simulink model "c00002M_harness"  (R2018a)
settings: Solver=FixedStepAuto  StartTime=0.0  StopTime=300  FixedStep=0.1  RelTol=1e-3
undefined symbols (not defined in the file): A1, hmax, R1, R2, sigbuilder_block, TempThreshold
(part 5 of 14)

== system c00002M_harness/M075/Tank3 ==
  CT3 : Inport
  MR3 : Inport  Port=2
  T3 : Inport  Port=3
  EB3 : Inport  Port=4
  Control : Subsystem
  Memory : Memory
  TankModel : Subsystem
  LL3 : Outport
  wires:
  TankModel/1(LiquidLevel) -> Memory/1, LL3/1
  Control/2(LiquidOut) -> TankModel/2(LiquidOut)
  Memory/1 -> Control/5(LiquidLevel)
  MR3/1 -> Control/2(ManualReference)
  CT3/1 -> Control/1(ControlType)
  EB3/1 -> Control/3(EmergencyButton)
  T3/1 -> Control/4(Temperature)
  Control/1(LiquidIn) -> TankModel/1(LiquidIn)

== system c00002M_harness/M076/Tank1 ==
  CT1 : Inport
  MR1 : Inport  Port=2
  T1 : Inport  Port=3
  EB1 : Inport  Port=4
  Control : Subsystem
  Memory : Memory
  TankModel : Subsystem
  LL1 : Outport
  wires:
  TankModel/1(LiquidLevel) -> Memory/1, LL1/1
  Control/2(LiquidOut) -> TankModel/2(LiquidOut)
  Memory/1 -> Control/5(LiquidLevel)
  MR1/1 -> Control/2(ManualReference)
  CT1/1 -> Control/1(ControlType)
  EB1/1 -> Control/3(EmergencyButton)
  T1/1 -> Control/4(Temperature)
  Control/1(LiquidIn) -> TankModel/1(LiquidIn)

== system c00002M_harness/M076/Tank3 ==
  CT3 : Inport
  MR3 : Inport  Port=2
  T3 : Inport  Port=3
  EB3 : Inport  Port=4
  Control : Subsystem
  Memory : Memory
  TankModel : Subsystem
  LL3 : Outport
  wires:
  TankModel/1(LiquidLevel) -> Memory/1, LL3/1
  Control/2(LiquidOut) -> TankModel/2(LiquidOut)
  Memory/1 -> Control/5(LiquidLevel)
  MR3/1 -> Control/2(ManualReference)
  CT3/1 -> Control/1(ControlType)
  EB3/1 -> Control/3(EmergencyButton)
  T3/1 -> Control/4(Temperature)
  Control/1(LiquidIn) -> TankModel/1(LiquidIn)

== system c00002M_harness/M077/Tank1 ==
  CT1 : Inport
  MR1 : Inport  Port=2
  T1 : Inport  Port=3
  EB1 : Inport  Port=4
  Control : Subsystem
  Memory : Memory
  TankModel : Subsystem
  LL1 : Outport
  wires:
  TankModel/1(LiquidLevel) -> Memory/1, LL1/1
  Control/2(LiquidOut) -> TankModel/2(LiquidOut)
  Memory/1 -> Control/5(LiquidLevel)
  MR1/1 -> Control/2(ManualReference)
  CT1/1 -> Control/1(ControlType)
  EB1/1 -> Control/3(EmergencyButton)
  T1/1 -> Control/4(Temperature)
  Control/1(LiquidIn) -> TankModel/1(LiquidIn)

== system c00002M_harness/M077/Tank3 ==
  CT3 : Inport
  MR3 : Inport  Port=2
  T3 : Inport  Port=3
  EB3 : Inport  Port=4
  Control : Subsystem
  Memory : Memory
  TankModel : Subsystem
  LL3 : Outport
  wires:
  TankModel/1(LiquidLevel) -> Memory/1, LL3/1
  Control/2(LiquidOut) -> TankModel/2(LiquidOut)
  Memory/1 -> Control/5(LiquidLevel)
  MR3/1 -> Control/2(ManualReference)
  CT3/1 -> Control/1(ControlType)
  EB3/1 -> Control/3(EmergencyButton)
  T3/1 -> Control/4(Temperature)
  Control/1(LiquidIn) -> TankModel/1(LiquidIn)

== system c00002M_harness/M078/Tank1 ==
  CT1 : Inport
  MR1 : Inport  Port=2
  T1 : Inport  Port=3
  EB1 : Inport  Port=4
  Control : Subsystem
  Memory : Memory
  TankModel : Subsystem
  LL1 : Outport
  wires:
  TankModel/1(LiquidLevel) -> Memory/1, LL1/1
  Control/2(LiquidOut) -> TankModel/2(LiquidOut)
  Memory/1 -> Control/5(LiquidLevel)
  MR1/1 -> Control/2(ManualReference)
  CT1/1 -> Control/1(ControlType)
  EB1/1 -> Control/3(EmergencyButton)
  T1/1 -> Control/4(Temperature)
  Control/1(LiquidIn) -> TankModel/1(LiquidIn)

== system c00002M_harness/M078/Tank3 ==
  CT3 : Inport
  MR3 : Inport  Port=2
  T3 : Inport  Port=3
  EB3 : Inport  Port=4
  Control : Subsystem
  Memory : Memory
  TankModel : Subsystem
  LL3 : Outport
  wires:
  TankModel/1(LiquidLevel) -> Memory/1, LL3/1
  Control/2(LiquidOut) -> TankModel/2(LiquidOut)
  Memory/1 -> Control/5(LiquidLevel)
  MR3/1 -> Control/2(ManualReference)
  CT3/1 -> Control/1(ControlType)
  EB3/1 -> Control/3(EmergencyButton)
  T3/1 -> Control/4(Temperature)
  Control/1(LiquidIn) -> TankModel/1(LiquidIn)

== system c00002M_harness/M079/Tank1 ==
  CT1 : Inport
  MR1 : Inport  Port=2
  T1 : Inport  Port=3
  EB1 : Inport  Port=4
  Control : Subsystem
  Memory : Memory
  TankModel : Subsystem
  LL1 : Outport
  wires:
  TankModel/1(LiquidLevel) -> Memory/1, LL1/1
  Control/2(LiquidOut) -> TankModel/2(LiquidOut)
  Memory/1 -> Control/5(LiquidLevel)
  MR1/1 -> Control/2(ManualReference)
  CT1/1 -> Control/1(ControlType)
  EB1/1 -> Control/3(EmergencyButton)
  T1/1 -> Control/4(Temperature)
  Control/1(LiquidIn) -> TankModel/1(LiquidIn)

== system c00002M_harness/M079/Tank3 ==
  CT3 : Inport
  MR3 : Inport  Port=2
  T3 : Inport  Port=3
  EB3 : Inport  Port=4
  Control : Subsystem
  Memory : Memory
  TankModel : Subsystem
  LL3 : Outport
  wires:
  TankModel/1(LiquidLevel) -> Memory/1, LL3/1
  Control/2(LiquidOut) -> TankModel/2(LiquidOut)
  Memory/1 -> Control/5(LiquidLevel)
  MR3/1 -> Control/2(ManualReference)
  CT3/1 -> Control/1(ControlType)
  EB3/1 -> Control/3(EmergencyButton)
  T3/1 -> Control/4(Temperature)
  Control/1(LiquidIn) -> TankModel/1(LiquidIn)

== system c00002M_harness/M080/Tank1 ==
  CT1 : Inport
  MR1 : Inport  Port=2
  T1 : Inport  Port=3
  EB1 : Inport  Port=4
  Control : Subsystem
  Memory : Memory
  TankModel : Subsystem
  LL1 : Outport
  wires:
  TankModel/1(LiquidLevel) -> Memory/1, LL1/1
  Control/2(LiquidOut) -> TankModel/2(LiquidOut)
  Memory/1 -> Control/5(LiquidLevel)
  MR1/1 -> Control/2(ManualReference)
  CT1/1 -> Control/1(ControlType)
  EB1/1 -> Control/3(EmergencyButton)
  T1/1 -> Control/4(Temperature)
  Control/1(LiquidIn) -> TankModel/1(LiquidIn)

== system c00002M_harness/M080/Tank3 ==
  CT3 : Inport
  MR3 : Inport  Port=2
  T3 : Inport  Port=3
  EB3 : Inport  Port=4
  Control : Subsystem
  Memory : Memory
  TankModel : Subsystem
  LL3 : Outport
  wires:
  TankModel/1(LiquidLevel) -> Memory/1, LL3/1
  Control/2(LiquidOut) -> TankModel/2(LiquidOut)
  Memory/1 -> Control/5(LiquidLevel)
  MR3/1 -> Control/2(ManualReference)
  CT3/1 -> Control/1(ControlType)
  EB3/1 -> Control/3(EmergencyButton)
  T3/1 -> Control/4(Temperature)
  Control/1(LiquidIn) -> TankModel/1(LiquidIn)

== system c00002M_harness/M081/Tank1 ==
  CT1 : Inport
  MR1 : Inport  Port=2
  T1 : Inport  Port=3
  EB1 : Inport  Port=4
  Control : Subsystem
  Memory : Memory
  TankModel : Subsystem
  LL1 : Outport
  wires:
  TankModel/1(LiquidLevel) -> Memory/1, LL1/1
  Control/2(LiquidOut) -> TankModel/2(LiquidOut)
  Memory/1 -> Control/5(LiquidLevel)
  MR1/1 -> Control/2(ManualReference)
  CT1/1 -> Control/1(ControlType)
  EB1/1 -> Control/3(EmergencyButton)
  T1/1 -> Control/4(Temperature)
  Control/1(LiquidIn) -> TankModel/1(LiquidIn)

== system c00002M_harness/M081/Tank3 ==
  CT3 : Inport
  MR3 : Inport  Port=2
  T3 : Inport  Port=3
  EB3 : Inport  Port=4
  Control : Subsystem
  Memory : Memory
  TankModel : Subsystem
  LL3 : Outport
  wires:
  TankModel/1(LiquidLevel) -> Memory/1, LL3/1
  Control/2(LiquidOut) -> TankModel/2(LiquidOut)
  Memory/1 -> Control/5(LiquidLevel)
  MR3/1 -> Control/2(ManualReference)
  CT3/1 -> Control/1(ControlType)
  EB3/1 -> Control/3(EmergencyButton)
  T3/1 -> Control/4(Temperature)
  Control/1(LiquidIn) -> TankModel/1(LiquidIn)

== system c00002M_harness/M082/Tank1 ==
  CT1 : Inport
  MR1 : Inport  Port=2
  T1 : Inport  Port=3
  EB1 : Inport  Port=4
  Control : Subsystem
  Memory : Memory
  TankModel : Subsystem
  LL1 : Outport
  wires:
  TankModel/1(LiquidLevel) -> Memory/1, LL1/1
  Control/2(LiquidOut) -> TankModel/2(LiquidOut)
  Memory/1 -> Control/5(LiquidLevel)
  MR1/1 -> Control/2(ManualReference)
  CT1/1 -> Control/1(ControlType)
  EB1/1 -> Control/3(EmergencyButton)
  T1/1 -> Control/4(Temperature)
  Control/1(LiquidIn) -> TankModel/1(LiquidIn)

== system c00002M_harness/M082/Tank3 ==
  CT3 : Inport
  MR3 : Inport  Port=2
  T3 : Inport  Port=3
  EB3 : Inport  Port=4
  Control : Subsystem
  Memory : Memory
  TankModel : Subsystem
  LL3 : Outport
  wires:
  TankModel/1(LiquidLevel) -> Memory/1, LL3/1
  Control/2(LiquidOut) -> TankModel/2(LiquidOut)
  Memory/1 -> Control/5(LiquidLevel)
  MR3/1 -> Control/2(ManualReference)
  CT3/1 -> Control/1(ControlType)
  EB3/1 -> Control/3(EmergencyButton)
  T3/1 -> Control/4(Temperature)
  Control/1(LiquidIn) -> TankModel/1(LiquidIn)

== system c00002M_harness/M165/Tank1 ==
  CT1 : Inport
  MR1 : Inport  Port=2
  T1 : Inport  Port=3
  EB1 : Inport  Port=4
  Control : Subsystem
  Memory : Memory
  TankModel : Subsystem
  LL1 : Outport
  wires:
  TankModel/1(LiquidLevel) -> Memory/1, LL1/1
  Control/2(LiquidOut) -> TankModel/2(LiquidOut)
  Memory/1 -> Control/5(LiquidLevel)
  MR1/1 -> Control/2(ManualReference)
  CT1/1 -> Control/1(ControlType)
  EB1/1 -> Control/3(EmergencyButton)
  T1/1 -> Control/4(Temperature)
  Control/1(LiquidIn) -> TankModel/1(LiquidIn)

== system c00002M_harness/M165/Tank3 ==
  CT3 : Inport
  MR3 : Inport  Port=2
  T3 : Inport  Port=3
  EB3 : Inport  Port=4
  Control : Subsystem
  Memory : Memory
  TankModel : Subsystem
  LL3 : Outport
  wires:
  TankModel/1(LiquidLevel) -> Memory/1, LL3/1
  Control/2(LiquidOut) -> TankModel/2(LiquidOut)
  Memory/1 -> Control/5(LiquidLevel)
  MR3/1 -> Control/2(ManualReference)
  CT3/1 -> Control/1(ControlType)
  EB3/1 -> Control/3(EmergencyButton)
  T3/1 -> Control/4(Temperature)
  Control/1(LiquidIn) -> TankModel/1(LiquidIn)

== system c00002M_harness/M166/Tank1 ==
  CT1 : Inport
  MR1 : Inport  Port=2
  T1 : Inport  Port=3
  EB1 : Inport  Port=4
  Control : Subsystem
  Memory : Memory
  TankModel : Subsystem
  LL1 : Outport
  wires:
  TankModel/1(LiquidLevel) -> Memory/1, LL1/1
  Control/2(LiquidOut) -> TankModel/2(LiquidOut)
  Memory/1 -> Control/5(LiquidLevel)
  MR1/1 -> Control/2(ManualReference)
  CT1/1 -> Control/1(ControlType)
  EB1/1 -> Control/3(EmergencyButton)
  T1/1 -> Control/4(Temperature)
  Control/1(LiquidIn) -> TankModel/1(LiquidIn)

== system c00002M_harness/M166/Tank3 ==
  CT3 : Inport
  MR3 : Inport  Port=2
  T3 : Inport  Port=3
  EB3 : Inport  Port=4
  Control : Subsystem
  Memory : Memory
  TankModel : Subsystem
  LL3 : Outport
  wires:
  TankModel/1(LiquidLevel) -> Memory/1, LL3/1
  Control/2(LiquidOut) -> TankModel/2(LiquidOut)
  Memory/1 -> Control/5(LiquidLevel)
  MR3/1 -> Control/2(ManualReference)
  CT3/1 -> Control/1(ControlType)
  EB3/1 -> Control/3(EmergencyButton)
  T3/1 -> Control/4(Temperature)
  Control/1(LiquidIn) -> TankModel/1(LiquidIn)

== system c00002M_harness/M167/Tank1 ==
  CT1 : Inport
  MR1 : Inport  Port=2
  T1 : Inport  Port=3
  EB1 : Inport  Port=4
  Control : Subsystem
  Memory : Memory
  TankModel : Subsystem
  LL1 : Outport
  wires:
  TankModel/1(LiquidLevel) -> Memory/1, LL1/1
  Control/2(LiquidOut) -> TankModel/2(LiquidOut)
  Memory/1 -> Control/5(LiquidLevel)
  MR1/1 -> Control/2(ManualReference)
  CT1/1 -> Control/1(ControlType)
  EB1/1 -> Control/3(EmergencyButton)
  T1/1 -> Control/4(Temperature)
  Control/1(LiquidIn) -> TankModel/1(LiquidIn)

== system c00002M_harness/M167/Tank3 ==
  CT3 : Inport
  MR3 : Inport  Port=2
  T3 : Inport  Port=3
  EB3 : Inport  Port=4
  Control : Subsystem
  Memory : Memory
  TankModel : Subsystem
  LL3 : Outport
  wires:
  TankModel/1(LiquidLevel) -> Memory/1, LL3/1
  Control/2(LiquidOut) -> TankModel/2(LiquidOut)
  Memory/1 -> Control/5(LiquidLevel)
  MR3/1 -> Control/2(ManualReference)
  CT3/1 -> Control/1(ControlType)
  EB3/1 -> Control/3(EmergencyButton)
  T3/1 -> Control/4(Temperature)
  Control/1(LiquidIn) -> TankModel/1(LiquidIn)

== system c00002M_harness/M168/Tank1 ==
  CT1 : Inport
  MR1 : Inport  Port=2
  T1 : Inport  Port=3
  EB1 : Inport  Port=4
  Control : Subsystem
  Memory : Memory
  TankModel : Subsystem
  LL1 : Outport
  wires:
  TankModel/1(LiquidLevel) -> Memory/1, LL1/1
  Control/2(LiquidOut) -> TankModel/2(LiquidOut)
  Memory/1 -> Control/5(LiquidLevel)
  MR1/1 -> Control/2(ManualReference)
  CT1/1 -> Control/1(ControlType)
  EB1/1 -> Control/3(EmergencyButton)
  T1/1 -> Control/4(Temperature)
  Control/1(LiquidIn) -> TankModel/1(LiquidIn)

== system c00002M_harness/M168/Tank3 ==
  CT3 : Inport
  MR3 : Inport  Port=2
  T3 : Inport  Port=3
  EB3 : Inport  Port=4
  Control : Subsystem
  Memory : Memory
  TankModel : Subsystem
  LL3 : Outport
  wires:
  TankModel/1(LiquidLevel) -> Memory/1, LL3/1
  Control/2(LiquidOut) -> TankModel/2(LiquidOut)
  Memory/1 -> Control/5(LiquidLevel)
  MR3/1 -> Control/2(ManualReference)
  CT3/1 -> Control/1(ControlType)
  EB3/1 -> Control/3(EmergencyButton)
  T3/1 -> Control/4(Temperature)
  Control/1(LiquidIn) -> TankModel/1(LiquidIn)

== system c00002M_harness/M210/Tank1 ==
  CT1 : Inport
  MR1 : Inport  Port=2
  T1 : Inport  Port=3
  EB1 : Inport  Port=4
  Control : Subsystem
  Memory : Memory
  TankModel : Subsystem
  LL1 : Outport
  wires:
  TankModel/1(LiquidLevel) -> Memory/1, LL1/1
  Control/2(LiquidOut) -> TankModel/2(LiquidOut)
  Memory/1 -> Control/5(LiquidLevel)
  MR1/1 -> Control/2(ManualReference)
  CT1/1 -> Control/1(ControlType)
  EB1/1 -> Control/3(EmergencyButton)
  T1/1 -> Control/4(Temperature)
  Control/1(LiquidIn) -> TankModel/1(LiquidIn)

== system c00002M_harness/M210/Tank3 ==
  CT3 : Inport
  MR3 : Inport  Port=2
  T3 : Inport  Port=3
  EB3 : Inport  Port=4
  Control : Subsystem
  Memory : Memory
  TankModel : Subsystem
  LL3 : Outport
  wires:
  TankModel/1(LiquidLevel) -> Memory/1, LL3/1
  Control/2(LiquidOut) -> TankModel/2(LiquidOut)
  Memory/1 -> Control/5(LiquidLevel)
  MR3/1 -> Control/2(ManualReference)
  CT3/1 -> Control/1(ControlType)
  EB3/1 -> Control/3(EmergencyButton)
  T3/1 -> Control/4(Temperature)
  Control/1(LiquidIn) -> TankModel/1(LiquidIn)

== system c00002M_harness/M211/Tank1 ==
  CT1 : Inport
  MR1 : Inport  Port=2
  T1 : Inport  Port=3
  EB1 : Inport  Port=4
  Control : Subsystem
  Memory : Memory
  TankModel : Subsystem
  LL1 : Outport
  wires:
  TankModel/1(LiquidLevel) -> Memory/1, LL1/1
  Control/2(LiquidOut) -> TankModel/2(LiquidOut)
  Memory/1 -> Control/5(LiquidLevel)
  MR1/1 -> Control/2(ManualReference)
  CT1/1 -> Control/1(ControlType)
  EB1/1 -> Control/3(EmergencyButton)
  T1/1 -> Control/4(Temperature)
  Control/1(LiquidIn) -> TankModel/1(LiquidIn)

== system c00002M_harness/M211/Tank3 ==
  CT3 : Inport
  MR3 : Inport  Port=2
  T3 : Inport  Port=3
  EB3 : Inport  Port=4
  Control : Subsystem
  Memory : Memory
  TankModel : Subsystem
  LL3 : Outport
  wires:
  TankModel/1(LiquidLevel) -> Memory/1, LL3/1
  Control/2(LiquidOut) -> TankModel/2(LiquidOut)
  Memory/1 -> Control/5(LiquidLevel)
  MR3/1 -> Control/2(ManualReference)
  CT3/1 -> Control/1(ControlType)
  EB3/1 -> Control/3(EmergencyButton)
  T3/1 -> Control/4(Temperature)
  Control/1(LiquidIn) -> TankModel/1(LiquidIn)

== system c00002M_harness/M212/Tank1 ==
  CT1 : Inport
  MR1 : Inport  Port=2
  T1 : Inport  Port=3
  EB1 : Inport  Port=4
  Control : Subsystem
  Memory : Memory
  TankModel : Subsystem
  LL1 : Outport
  wires:
  TankModel/1(LiquidLevel) -> Memory/1, LL1/1
  Control/2(LiquidOut) -> TankModel/2(LiquidOut)
  Memory/1 -> Control/5(LiquidLevel)
  MR1/1 -> Control/2(ManualReference)
  CT1/1 -> Control/1(ControlType)
  EB1/1 -> Control/3(EmergencyButton)
  T1/1 -> Control/4(Temperature)
  Control/1(LiquidIn) -> TankModel/1(LiquidIn)

== system c00002M_harness/M212/Tank3 ==
  CT3 : Inport
  MR3 : Inport  Port=2
  T3 : Inport  Port=3
  EB3 : Inport  Port=4
  Control : Subsystem
  Memory : Memory
  TankModel : Subsystem
  LL3 : Outport
  wires:
  TankModel/1(LiquidLevel) -> Memory/1, LL3/1
  Control/2(LiquidOut) -> TankModel/2(LiquidOut)
  Memory/1 -> Control/5(LiquidLevel)
  MR3/1 -> Control/2(ManualReference)
  CT3/1 -> Control/1(ControlType)
  EB3/1 -> Control/3(EmergencyButton)
  T3/1 -> Control/4(Temperature)
  Control/1(LiquidIn) -> TankModel/1(LiquidIn)

== system c00002M_harness/M213/Tank1 ==
  CT1 : Inport
  MR1 : Inport  Port=2
  T1 : Inport  Port=3
  EB1 : Inport  Port=4
  Control : Subsystem
  Memory : Memory
  TankModel : Subsystem
  LL1 : Outport
  wires:
  TankModel/1(LiquidLevel) -> Memory/1, LL1/1
  Control/2(LiquidOut) -> TankModel/2(LiquidOut)
  Memory/1 -> Control/5(LiquidLevel)
  MR1/1 -> Control/2(ManualReference)
  CT1/1 -> Control/1(ControlType)
  EB1/1 -> Control/3(EmergencyButton)
  T1/1 -> Control/4(Temperature)
  Control/1(LiquidIn) -> TankModel/1(LiquidIn)

== system c00002M_harness/M213/Tank3 ==
  CT3 : Inport
  MR3 : Inport  Port=2
  T3 : Inport  Port=3
  EB3 : Inport  Port=4
  Control : Subsystem
  Memory : Memory
  TankModel : Subsystem
  LL3 : Outport
  wires:
  TankModel/1(LiquidLevel) -> Memory/1, LL3/1
  Control/2(LiquidOut) -> TankModel/2(LiquidOut)
  Memory/1 -> Control/5(LiquidLevel)
  MR3/1 -> Control/2(ManualReference)
  CT3/1 -> Control/1(ControlType)
  EB3/1 -> Control/3(EmergencyButton)
  T3/1 -> Control/4(Temperature)
  Control/1(LiquidIn) -> TankModel/1(LiquidIn)

== system c00002M_harness/M214/Tank1 ==
  CT1 : Inport
  MR1 : Inport  Port=2
  T1 : Inport  Port=3
  EB1 : Inport  Port=4
  Control : Subsystem
  Memory : Memory
  TankModel : Subsystem
  LL1 : Outport
  wires:
  TankModel/1(LiquidLevel) -> Memory/1, LL1/1
  Control/2(LiquidOut) -> TankModel/2(LiquidOut)
  Memory/1 -> Control/5(LiquidLevel)
  MR1/1 -> Control/2(ManualReference)
  CT1/1 -> Control/1(ControlType)
  EB1/1 -> Control/3(EmergencyButton)
  T1/1 -> Control/4(Temperature)
  Control/1(LiquidIn) -> TankModel/1(LiquidIn)

== system c00002M_harness/M214/Tank3 ==
  CT3 : Inport
  MR3 : Inport  Port=2
  T3 : Inport  Port=3
  EB3 : Inport  Port=4
  Control : Subsystem
  Memory : Memory
  TankModel : Subsystem
  LL3 : Outport
  wires:
  TankModel/1(LiquidLevel) -> Memory/1, LL3/1
  Control/2(LiquidOut) -> TankModel/2(LiquidOut)
  Memory/1 -> Control/5(LiquidLevel)
  MR3/1 -> Control/2(ManualReference)
  CT3/1 -> Control/1(ControlType)
  EB3/1 -> Control/3(EmergencyButton)
  T3/1 -> Control/4(Temperature)
  Control/1(LiquidIn) -> TankModel/1(LiquidIn)

== system c00002M_harness/M215/Tank1 ==
  CT1 : Inport
  MR1 : Inport  Port=2
  T1 : Inport  Port=3
  EB1 : Inport  Port=4
  Control : Subsystem
  Memory : Memory
  TankModel : Subsystem
  LL1 : Outport
  wires:
  TankModel/1(LiquidLevel) -> Memory/1, LL1/1
  Control/2(LiquidOut) -> TankModel/2(LiquidOut)
  Memory/1 -> Control/5(LiquidLevel)
  MR1/1 -> Control/2(ManualReference)
  CT1/1 -> Control/1(ControlType)
  EB1/1 -> Control/3(EmergencyButton)
  T1/1 -> Control/4(Temperature)
  Control/1(LiquidIn) -> TankModel/1(LiquidIn)

== system c00002M_harness/M215/Tank3 ==
  CT3 : Inport
  MR3 : Inport  Port=2
  T3 : Inport  Port=3
  EB3 : Inport  Port=4
  Control : Subsystem
  Memory : Memory
  TankModel : Subsystem
  LL3 : Outport
  wires:
  TankModel/1(LiquidLevel) -> Memory/1, LL3/1
  Control/2(LiquidOut) -> TankModel/2(LiquidOut)
  Memory/1 -> Control/5(LiquidLevel)
  MR3/1 -> Control/2(ManualReference)
  CT3/1 -> Control/1(ControlType)
  EB3/1 -> Control/3(EmergencyButton)
  T3/1 -> Control/4(Temperature)
  Control/1(LiquidIn) -> TankModel/1(LiquidIn)

== system c00002M_harness/M216/Tank1 ==
  CT1 : Inport
  MR1 : Inport  Port=2
  T1 : Inport  Port=3
  EB1 : Inport  Port=4
  Control : Subsystem
  Memory : Memory
  TankModel : Subsystem
  LL1 : Outport
  wires:
  TankModel/1(LiquidLevel) -> Memory/1, LL1/1
  Control/2(LiquidOut) -> TankModel/2(LiquidOut)
  Memory/1 -> Control/5(LiquidLevel)
  MR1/1 -> Control/2(ManualReference)
  CT1/1 -> Control/1(ControlType)
  EB1/1 -> Control/3(EmergencyButton)
  T1/1 -> Control/4(Temperature)
  Control/1(LiquidIn) -> TankModel/1(LiquidIn)

== system c00002M_harness/M216/Tank3 ==
  CT3 : Inport
  MR3 : Inport  Port=2
  T3 : Inport  Port=3
  EB3 : Inport  Port=4
  Control : Subsystem
  Memory : Memory
  TankModel : Subsystem
  LL3 : Outport
  wires:
  TankModel/1(LiquidLevel) -> Memory/1, LL3/1
  Control/2(LiquidOut) -> TankModel/2(LiquidOut)
  Memory/1 -> Control/5(LiquidLevel)
  MR3/1 -> Control/2(ManualReference)
  CT3/1 -> Control/1(ControlType)
  EB3/1 -> Control/3(EmergencyButton)
  T3/1 -> Control/4(Temperature)
  Control/1(LiquidIn) -> TankModel/1(LiquidIn)

== system c00002M_harness/M217/Tank1 ==
  CT1 : Inport
  MR1 : Inport  Port=2
  T1 : Inport  Port=3
  EB1 : Inport  Port=4
  Control : Subsystem
  Memory : Memory
  TankModel : Subsystem
  LL1 : Outport
  wires:
  TankModel/1(LiquidLevel) -> Memory/1, LL1/1
  Control/2(LiquidOut) -> TankModel/2(LiquidOut)
  Memory/1 -> Control/5(LiquidLevel)
  MR1/1 -> Control/2(ManualReference)
  CT1/1 -> Control/1(ControlType)
  EB1/1 -> Control/3(EmergencyButton)
  T1/1 -> Control/4(Temperature)
  Control/1(LiquidIn) -> TankModel/1(LiquidIn)

== system c00002M_harness/M217/Tank3 ==
  CT3 : Inport
  MR3 : Inport  Port=2
  T3 : Inport  Port=3
  EB3 : Inport  Port=4
  Control : Subsystem
  Memory : Memory
  TankModel : Subsystem
  LL3 : Outport
  wires:
  TankModel/1(LiquidLevel) -> Memory/1, LL3/1
  Control/2(LiquidOut) -> TankModel/2(LiquidOut)
  Memory/1 -> Control/5(LiquidLevel)
  MR3/1 -> Control/2(ManualReference)
  CT3/1 -> Control/1(ControlType)
  EB3/1 -> Control/3(EmergencyButton)
  T3/1 -> Control/4(Temperature)
  Control/1(LiquidIn) -> TankModel/1(LiquidIn)

== system c00002M_harness/M218/Tank1 ==
  CT1 : Inport
  MR1 : Inport  Port=2
  T1 : Inport  Port=3
  EB1 : Inport  Port=4
  Control : Subsystem
  Memory : Memory
  TankModel : Subsystem
  LL1 : Outport
  wires:
  TankModel/1(LiquidLevel) -> Memory/1, LL1/1
  Control/2(LiquidOut) -> TankModel/2(LiquidOut)
  Memory/1 -> Control/5(LiquidLevel)
  MR1/1 -> Control/2(ManualReference)
  CT1/1 -> Control/1(ControlType)
  EB1/1 -> Control/3(EmergencyButton)
  T1/1 -> Control/4(Temperature)
  Control/1(LiquidIn) -> TankModel/1(LiquidIn)

== system c00002M_harness/M218/Tank3 ==
  CT3 : Inport
  MR3 : Inport  Port=2
  T3 : Inport  Port=3
  EB3 : Inport  Port=4
  Control : Subsystem
  Memory : Memory
  TankModel : Subsystem
  LL3 : Outport
  wires:
  TankModel/1(LiquidLevel) -> Memory/1, LL3/1
  Control/2(LiquidOut) -> TankModel/2(LiquidOut)
  Memory/1 -> Control/5(LiquidLevel)
  MR3/1 -> Control/2(ManualReference)
  CT3/1 -> Control/1(ControlType)
  EB3/1 -> Control/3(EmergencyButton)
  T3/1 -> Control/4(Temperature)
  Control/1(LiquidIn) -> TankModel/1(LiquidIn)

== system c00002M_harness/M219/Tank1 ==
  CT1 : Inport
  MR1 : Inport  Port=2
  T1 : Inport  Port=3
  EB1 : Inport  Port=4
  Control : Subsystem
  Memory : Memory
  TankModel : Subsystem
  LL1 : Outport
  wires:
  TankModel/1(LiquidLevel) -> Memory/1, LL1/1
  Control/2(LiquidOut) -> TankModel/2(LiquidOut)
  Memory/1 -> Control/5(LiquidLevel)
  MR1/1 -> Control/2(ManualReference)
  CT1/1 -> Control/1(ControlType)
  EB1/1 -> Control/3(EmergencyButton)
  T1/1 -> Control/4(Temperature)
  Control/1(LiquidIn) -> TankModel/1(LiquidIn)

== system c00002M_harness/M219/Tank3 ==
  CT3 : Inport
  MR3 : Inport  Port=2
  T3 : Inport  Port=3
  EB3 : Inport  Port=4
  Control : Subsystem
  Memory : Memory
  TankModel : Subsystem
  LL3 : Outport
  wires:
  TankModel/1(LiquidLevel) -> Memory/1, LL3/1
  Control/2(LiquidOut) -> TankModel/2(LiquidOut)
  Memory/1 -> Control/5(LiquidLevel)
  MR3/1 -> Control/2(ManualReference)
  CT3/1 -> Control/1(ControlType)
  EB3/1 -> Control/3(EmergencyButton)
  T3/1 -> Control/4(Temperature)
  Control/1(LiquidIn) -> TankModel/1(LiquidIn)

== system c00002M_harness/M220/Tank1 ==
  CT1 : Inport
  MR1 : Inport  Port=2
  T1 : Inport  Port=3
  EB1 : Inport  Port=4
  Control : Subsystem
  Memory : Memory
  TankModel : Subsystem
  LL1 : Outport
  wires:
  TankModel/1(LiquidLevel) -> Memory/1, LL1/1
  Control/2(LiquidOut) -> TankModel/2(LiquidOut)
  Memory/1 -> Control/5(LiquidLevel)
  MR1/1 -> Control/2(ManualReference)
  CT1/1 -> Control/1(ControlType)
  EB1/1 -> Control/3(EmergencyButton)
  T1/1 -> Control/4(Temperature)
  Control/1(LiquidIn) -> TankModel/1(LiquidIn)

== system c00002M_harness/M220/Tank3 ==
  CT3 : Inport
  MR3 : Inport  Port=2
  T3 : Inport  Port=3
  EB3 : Inport  Port=4
  Control : Subsystem
  Memory : Memory
  TankModel : Subsystem
  LL3 : Outport
  wires:
  TankModel/1(LiquidLevel) -> Memory/1, LL3/1
  Control/2(LiquidOut) -> TankModel/2(LiquidOut)
  Memory/1 -> Control/5(LiquidLevel)
  MR3/1 -> Control/2(ManualReference)
  CT3/1 -> Control/1(ControlType)
  EB3/1 -> Control/3(EmergencyButton)
  T3/1 -> Control/4(Temperature)
  Control/1(LiquidIn) -> TankModel/1(LiquidIn)

== system c00002M_harness/M221/Tank1 ==
  CT1 : Inport
  MR1 : Inport  Port=2
  T1 : Inport  Port=3
  EB1 : Inport  Port=4
  Control : Subsystem
  Memory : Memory
  TankModel : Subsystem
  LL1 : Outport
  wires:
  TankModel/1(LiquidLevel) -> Memory/1, LL1/1
  Control/2(LiquidOut) -> TankModel/2(LiquidOut)
  Memory/1 -> Control/5(LiquidLevel)
  MR1/1 -> Control/2(ManualReference)
  CT1/1 -> Control/1(ControlType)
  EB1/1 -> Control/3(EmergencyButton)
  T1/1 -> Control/4(Temperature)
  Control/1(LiquidIn) -> TankModel/1(LiquidIn)

== system c00002M_harness/M221/Tank3 ==
  CT3 : Inport
  MR3 : Inport  Port=2
  T3 : Inport  Port=3
  EB3 : Inport  Port=4
  Control : Subsystem
  Memory : Memory
  TankModel : Subsystem
  LL3 : Outport
  wires:
  TankModel/1(LiquidLevel) -> Memory/1, LL3/1
  Control/2(LiquidOut) -> TankModel/2(LiquidOut)
  Memory/1 -> Control/5(LiquidLevel)
  MR3/1 -> Control/2(ManualReference)
  CT3/1 -> Control/1(ControlType)
  EB3/1 -> Control/3(EmergencyButton)
  T3/1 -> Control/4(Temperature)
  Control/1(LiquidIn) -> TankModel/1(LiquidIn)

== system c00002M_harness/M222/Tank1 ==
  CT1 : Inport
  MR1 : Inport  Port=2
  T1 : Inport  Port=3
  EB1 : Inport  Port=4
  Control : Subsystem
  Memory : Memory
  TankModel : Subsystem
  LL1 : Outport
  wires:
  TankModel/1(LiquidLevel) -> Memory/1, LL1/1
  Control/2(LiquidOut) -> TankModel/2(LiquidOut)
  Memory/1 -> Control/5(LiquidLevel)
  MR1/1 -> Control/2(ManualReference)
  CT1/1 -> Control/1(ControlType)
  EB1/1 -> Control/3(EmergencyButton)
  T1/1 -> Control/4(Temperature)
  Control/1(LiquidIn) -> TankModel/1(LiquidIn)

== system c00002M_harness/M222/Tank3 ==
  CT3 : Inport
  MR3 : Inport  Port=2
  T3 : Inport  Port=3
  EB3 : Inport  Port=4
  Control : Subsystem
  Memory : Memory
  TankModel : Subsystem
  LL3 : Outport
  wires:
  TankModel/1(LiquidLevel) -> Memory/1, LL3/1
  Control/2(LiquidOut) -> TankModel/2(LiquidOut)
  Memory/1 -> Control/5(LiquidLevel)
  MR3/1 -> Control/2(ManualReference)
  CT3/1 -> Control/1(ControlType)
  EB3/1 -> Control/3(EmergencyButton)
  T3/1 -> Control/4(Temperature)
  Control/1(LiquidIn) -> TankModel/1(LiquidIn)

== system c00002M_harness/M223/Tank1 ==
  CT1 : Inport
  MR1 : Inport  Port=2
  T1 : Inport  Port=3
  EB1 : Inport  Port=4
  Control : Subsystem
  Memory : Memory
  TankModel : Subsystem
  LL1 : Outport
  wires:
  TankModel/1(LiquidLevel) -> Memory/1, LL1/1
  Control/2(LiquidOut) -> TankModel/2(LiquidOut)
  Memory/1 -> Control/5(LiquidLevel)
  MR1/1 -> Control/2(ManualReference)
  CT1/1 -> Control/1(ControlType)
  EB1/1 -> Control/3(EmergencyButton)
  T1/1 -> Control/4(Temperature)
  Control/1(LiquidIn) -> TankModel/1(LiquidIn)

== system c00002M_harness/M223/Tank3 ==
  CT3 : Inport
  MR3 : Inport  Port=2
  T3 : Inport  Port=3
  EB3 : Inport  Port=4
  Control : Subsystem
  Memory : Memory
  TankModel : Subsystem
  LL3 : Outport
  wires:
  TankModel/1(LiquidLevel) -> Memory/1, LL3/1
  Control/2(LiquidOut) -> TankModel/2(LiquidOut)
  Memory/1 -> Control/5(LiquidLevel)
  MR3/1 -> Control/2(ManualReference)
  CT3/1 -> Control/1(ControlType)
  EB3/1 -> Control/3(EmergencyButton)
  T3/1 -> Control/4(Temperature)
  Control/1(LiquidIn) -> TankModel/1(LiquidIn)

== system c00002M_harness/M224/Tank1 ==
  CT1 : Inport
  MR1 : Inport  Port=2
  T1 : Inport  Port=3
  EB1 : Inport  Port=4
  Control : Subsystem
  Memory : Memory
  TankModel : Subsystem
  LL1 : Outport
  wires:
  TankModel/1(LiquidLevel) -> Memory/1, LL1/1
  Control/2(LiquidOut) -> TankModel/2(LiquidOut)
  Memory/1 -> Control/5(LiquidLevel)
  MR1/1 -> Control/2(ManualReference)
  CT1/1 -> Control/1(ControlType)
  EB1/1 -> Control/3(EmergencyButton)
  T1/1 -> Control/4(Temperature)
  Control/1(LiquidIn) -> TankModel/1(LiquidIn)

== system c00002M_harness/M224/Tank3 ==
  CT3 : Inport
  MR3 : Inport  Port=2
  T3 : Inport  Port=3
  EB3 : Inport  Port=4
  Control : Subsystem
  Memory : Memory
  TankModel : Subsystem
  LL3 : Outport
  wires:
  TankModel/1(LiquidLevel) -> Memory/1, LL3/1
  Control/2(LiquidOut) -> TankModel/2(LiquidOut)
  Memory/1 -> Control/5(LiquidLevel)
  MR3/1 -> Control/2(ManualReference)
  CT3/1 -> Control/1(ControlType)
  EB3/1 -> Control/3(EmergencyButton)
  T3/1 -> Control/4(Temperature)
  Control/1(LiquidIn) -> TankModel/1(LiquidIn)

== system c00002M_harness/M225/Tank1 ==
  CT1 : Inport
  MR1 : Inport  Port=2
  T1 : Inport  Port=3
  EB1 : Inport  Port=4
  Control : Subsystem
  Memory : Memory
  TankModel : Subsystem
  LL1 : Outport
  wires:
  TankModel/1(LiquidLevel) -> Memory/1, LL1/1
  Control/2(LiquidOut) -> TankModel/2(LiquidOut)
  Memory/1 -> Control/5(LiquidLevel)
  MR1/1 -> Control/2(ManualReference)
  CT1/1 -> Control/1(ControlType)
  EB1/1 -> Control/3(EmergencyButton)
  T1/1 -> Control/4(Temperature)
  Control/1(LiquidIn) -> TankModel/1(LiquidIn)

== system c00002M_harness/M225/Tank3 ==
  CT3 : Inport
  MR3 : Inport  Port=2
  T3 : Inport  Port=3
  EB3 : Inport  Port=4
  Control : Subsystem
  Memory : Memory
  TankModel : Subsystem
  LL3 : Outport
  wires:
  TankModel/1(LiquidLevel) -> Memory/1, LL3/1
  Control/2(LiquidOut) -> TankModel/2(LiquidOut)
  Memory/1 -> Control/5(LiquidLevel)
  MR3/1 -> Control/2(ManualReference)
  CT3/1 -> Control/1(ControlType)
  EB3/1 -> Control/3(EmergencyButton)
  T3/1 -> Control/4(Temperature)
  Control/1(LiquidIn) -> TankModel/1(LiquidIn)

== system c00002M_harness/M233/Tank1 ==
  CT1 : Inport
  MR1 : Inport  Port=2
  T1 : Inport  Port=3
  EB1 : Inport  Port=4
  Control : Subsystem
  Memory : Memory
  TankModel : Subsystem
  LL1 : Outport
  wires:
  TankModel/1(LiquidLevel) -> Memory/1, LL1/1
  Control/2(LiquidOut) -> TankModel/2(LiquidOut)
  Memory/1 -> Control/5(LiquidLevel)
  MR1/1 -> Control/2(ManualReference)
  CT1/1 -> Control/1(ControlType)
  EB1/1 -> Control/3(EmergencyButton)
  T1/1 -> Control/4(Temperature)
  Control/1(LiquidIn) -> TankModel/1(LiquidIn)

== system c00002M_harness/M233/Tank3 ==
  CT3 : Inport
  MR3 : Inport  Port=2
  T3 : Inport  Port=3
  EB3 : Inport  Port=4
  Control : Subsystem
  Memory : Memory
  TankModel : Subsystem
  LL3 : Outport
  wires:
  TankModel/1(LiquidLevel) -> Memory/1, LL3/1
  Control/2(LiquidOut) -> TankModel/2(LiquidOut)
  Memory/1 -> Control/5(LiquidLevel)
  MR3/1 -> Control/2(ManualReference)
  CT3/1 -> Control/1(ControlType)
  EB3/1 -> Control/3(EmergencyButton)
  T3/1 -> Control/4(Temperature)
  Control/1(LiquidIn) -> TankModel/1(LiquidIn)

== system c00002M_harness/M234/Tank1 ==
  CT1 : Inport
  MR1 : Inport  Port=2
  T1 : Inport  Port=3
  EB1 : Inport  Port=4
  Control : Subsystem
  Memory : Memory
  TankModel : Subsystem
  LL1 : Outport
  wires:
  TankModel/1(LiquidLevel) -> Memory/1, LL1/1
  Control/2(LiquidOut) -> TankModel/2(LiquidOut)
  Memory/1 -> Control/5(LiquidLevel)
  MR1/1 -> Control/2(ManualReference)
  CT1/1 -> Control/1(ControlType)
  EB1/1 -> Control/3(EmergencyButton)
  T1/1 -> Control/4(Temperature)
  Control/1(LiquidIn) -> TankModel/1(LiquidIn)

== system c00002M_harness/M234/Tank3 ==
  CT3 : Inport
  MR3 : Inport  Port=2
  T3 : Inport  Port=3
  EB3 : Inport  Port=4
  Control : Subsystem
  Memory : Memory
  TankModel : Subsystem
  LL3 : Outport
  wires:
  TankModel/1(LiquidLevel) -> Memory/1, LL3/1
  Control/2(LiquidOut) -> TankModel/2(LiquidOut)
  Memory/1 -> Control/5(LiquidLevel)
  MR3/1 -> Control/2(ManualReference)
  CT3/1 -> Control/1(ControlType)
  EB3/1 -> Control/3(EmergencyButton)
  T3/1 -> Control/4(Temperature)
  Control/1(LiquidIn) -> TankModel/1(LiquidIn)

== system c00002M_harness/M235/Tank1 ==
  CT1 : Inport
  MR1 : Inport  Port=2
  T1 : Inport  Port=3
  EB1 : Inport  Port=4
  Control : Subsystem
  Memory : Memory
  TankModel : Subsystem
  LL1 : Outport
  wires:
  TankModel/1(LiquidLevel) -> Memory/1, LL1/1
  Control/2(LiquidOut) -> TankModel/2(LiquidOut)
  Memory/1 -> Control/5(LiquidLevel)
  MR1/1 -> Control/2(ManualReference)
  CT1/1 -> Control/1(ControlType)
  EB1/1 -> Control/3(EmergencyButton)
  T1/1 -> Control/4(Temperature)
  Control/1(LiquidIn) -> TankModel/1(LiquidIn)

== system c00002M_harness/M235/Tank3 ==
  CT3 : Inport
  MR3 : Inport  Port=2
  T3 : Inport  Port=3
  EB3 : Inport  Port=4
  Control : Subsystem
  Memory : Memory
  TankModel : Subsystem
  LL3 : Outport
  wires:
  TankModel/1(LiquidLevel) -> Memory/1, LL3/1
  Control/2(LiquidOut) -> TankModel/2(LiquidOut)
  Memory/1 -> Control/5(LiquidLevel)
  MR3/1 -> Control/2(ManualReference)
  CT3/1 -> Control/1(ControlType)
  EB3/1 -> Control/3(EmergencyButton)
  T3/1 -> Control/4(Temperature)
  Control/1(LiquidIn) -> TankModel/1(LiquidIn)

== system c00002M_harness/M236/Tank1 ==
  CT1 : Inport
  MR1 : Inport  Port=2
  T1 : Inport  Port=3
  EB1 : Inport  Port=4
  Control : Subsystem
  Memory : Memory
  TankModel : Subsystem
  LL1 : Outport
  wires:
  TankModel/1(LiquidLevel) -> Memory/1, LL1/1
  Control/2(LiquidOut) -> TankModel/2(LiquidOut)
  Memory/1 -> Control/5(LiquidLevel)
  MR1/1 -> Control/2(ManualReference)
  CT1/1 -> Control/1(ControlType)
  EB1/1 -> Control/3(EmergencyButton)
  T1/1 -> Control/4(Temperature)
  Control/1(LiquidIn) -> TankModel/1(LiquidIn)

== system c00002M_harness/M236/Tank3 ==
  CT3 : Inport
  MR3 : Inport  Port=2
  T3 : Inport  Port=3
  EB3 : Inport  Port=4
  Control : Subsystem
  Memory : Memory
  TankModel : Subsystem
  LL3 : Outport
  wires:
  TankModel/1(LiquidLevel) -> Memory/1, LL3/1
  Control/2(LiquidOut) -> TankModel/2(LiquidOut)
  Memory/1 -> Control/5(LiquidLevel)
  MR3/1 -> Control/2(ManualReference)
  CT3/1 -> Control/1(ControlType)
  EB3/1 -> Control/3(EmergencyButton)
  T3/1 -> Control/4(Temperature)
  Control/1(LiquidIn) -> TankModel/1(LiquidIn)

== system c00002M_harness/M237/Tank1 ==
  CT1 : Inport
  MR1 : Inport  Port=2
  T1 : Inport  Port=3
  EB1 : Inport  Port=4
  Control : Subsystem
  Memory : Memory
  TankModel : Subsystem
  LL1 : Outport
  wires:
  TankModel/1(LiquidLevel) -> Memory/1, LL1/1
  Control/2(LiquidOut) -> TankModel/2(LiquidOut)
  Memory/1 -> Control/5(LiquidLevel)
  MR1/1 -> Control/2(ManualReference)
  CT1/1 -> Control/1(ControlType)
  EB1/1 -> Control/3(EmergencyButton)
  T1/1 -> Control/4(Temperature)
  Control/1(LiquidIn) -> TankModel/1(LiquidIn)

== system c00002M_harness/M237/Tank3 ==
  CT3 : Inport
  MR3 : Inport  Port=2
  T3 : Inport  Port=3
  EB3 : Inport  Port=4
  Control : Subsystem
  Memory : Memory
  TankModel : Subsystem
  LL3 : Outport
  wires:
  TankModel/1(LiquidLevel) -> Memory/1, LL3/1
  Control/2(LiquidOut) -> TankModel/2(LiquidOut)
  Memory/1 -> Control/5(LiquidLevel)
  MR3/1 -> Control/2(ManualReference)
  CT3/1 -> Control/1(ControlType)
  EB3/1 -> Control/3(EmergencyButton)
  T3/1 -> Control/4(Temperature)
  Control/1(LiquidIn) -> TankModel/1(LiquidIn)

== system c00002M_harness/M238/Tank1 ==
  CT1 : Inport
  MR1 : Inport  Port=2
  T1 : Inport  Port=3
  EB1 : Inport  Port=4
  Control : Subsystem
  Memory : Memory
  TankModel : Subsystem
  LL1 : Outport
  wires:
  TankModel/1(LiquidLevel) -> Memory/1, LL1/1
  Control/2(LiquidOut) -> TankModel/2(LiquidOut)
  Memory/1 -> Control/5(LiquidLevel)
  MR1/1 -> Control/2(ManualReference)
  CT1/1 -> Control/1(ControlType)
  EB1/1 -> Control/3(EmergencyButton)
  T1/1 -> Control/4(Temperature)
  Control/1(LiquidIn) -> TankModel/1(LiquidIn)

== system c00002M_harness/M238/Tank3 ==
  CT3 : Inport
  MR3 : Inport  Port=2
  T3 : Inport  Port=3
  EB3 : Inport  Port=4
  Control : Subsystem
  Memory : Memory
  TankModel : Subsystem
  LL3 : Outport
  wires:
  TankModel/1(LiquidLevel) -> Memory/1, LL3/1
  Control/2(LiquidOut) -> TankModel/2(LiquidOut)
  Memory/1 -> Control/5(LiquidLevel)
  MR3/1 -> Control/2(ManualReference)
  CT3/1 -> Control/1(ControlType)
  EB3/1 -> Control/3(EmergencyButton)
  T3/1 -> Control/4(Temperature)
  Control/1(LiquidIn) -> TankModel/1(LiquidIn)

== system c00002M_harness/M239/Tank1 ==
  CT1 : Inport
  MR1 : Inport  Port=2
  T1 : Inport  Port=3
  EB1 : Inport  Port=4
  Control : Subsystem
  Memory : Memory
  TankModel : Subsystem
  LL1 : Outport
  wires:
  TankModel/1(LiquidLevel) -> Memory/1, LL1/1
  Control/2(LiquidOut) -> TankModel/2(LiquidOut)
  Memory/1 -> Control/5(LiquidLevel)
  MR1/1 -> Control/2(ManualReference)
  CT1/1 -> Control/1(ControlType)
  EB1/1 -> Control/3(EmergencyButton)
  T1/1 -> Control/4(Temperature)
  Control/1(LiquidIn) -> TankModel/1(LiquidIn)

== system c00002M_harness/M239/Tank3 ==
  CT3 : Inport
  MR3 : Inport  Port=2
  T3 : Inport  Port=3
  EB3 : Inport  Port=4
  Control : Subsystem
  Memory : Memory
  TankModel : Subsystem
  LL3 : Outport
  wires:
  TankModel/1(LiquidLevel) -> Memory/1, LL3/1
  Control/2(LiquidOut) -> TankModel/2(LiquidOut)
  Memory/1 -> Control/5(LiquidLevel)
  MR3/1 -> Control/2(ManualReference)
  CT3/1 -> Control/1(ControlType)
  EB3/1 -> Control/3(EmergencyButton)
  T3/1 -> Control/4(Temperature)
  Control/1(LiquidIn) -> TankModel/1(LiquidIn)

== system c00002M_harness/M240/Tank1 ==
  CT1 : Inport
  MR1 : Inport  Port=2
  T1 : Inport  Port=3
  EB1 : Inport  Port=4
  Control : Subsystem
  Memory : Memory
  TankModel : Subsystem
  LL1 : Outport
  wires:
  TankModel/1(LiquidLevel) -> Memory/1, LL1/1
  Control/2(LiquidOut) -> TankModel/2(LiquidOut)
  Memory/1 -> Control/5(LiquidLevel)
  MR1/1 -> Control/2(ManualReference)
  CT1/1 -> Control/1(ControlType)
  EB1/1 -> Control/3(EmergencyButton)
  T1/1 -> Control/4(Temperature)
  Control/1(LiquidIn) -> TankModel/1(LiquidIn)

== system c00002M_harness/M240/Tank3 ==
  CT3 : Inport
  MR3 : Inport  Port=2
  T3 : Inport  Port=3
  EB3 : Inport  Port=4
  Control : Subsystem
  Memory : Memory
  TankModel : Subsystem
  LL3 : Outport
  wires:
  TankModel/1(LiquidLevel) -> Memory/1, LL3/1
  Control/2(LiquidOut) -> TankModel/2(LiquidOut)
  Memory/1 -> Control/5(LiquidLevel)
  MR3/1 -> Control/2(ManualReference)
  CT3/1 -> Control/1(ControlType)
  EB3/1 -> Control/3(EmergencyButton)
  T3/1 -> Control/4(Temperature)
  Control/1(LiquidIn) -> TankModel/1(LiquidIn)

== system c00002M_harness/M241/Tank1 ==
  CT1 : Inport
  MR1 : Inport  Port=2
  T1 : Inport  Port=3
  EB1 : Inport  Port=4
  Control : Subsystem
  Memory : Memory
  TankModel : Subsystem
  LL1 : Outport
  wires:
  TankModel/1(LiquidLevel) -> Memory/1, LL1/1
  Control/2(LiquidOut) -> TankModel/2(LiquidOut)
  Memory/1 -> Control/5(LiquidLevel)
  MR1/1 -> Control/2(ManualReference)
  CT1/1 -> Control/1(ControlType)
  EB1/1 -> Control/3(EmergencyButton)
  T1/1 -> Control/4(Temperature)
  Control/1(LiquidIn) -> TankModel/1(LiquidIn)

== system c00002M_harness/M241/Tank3 ==
  CT3 : Inport
  MR3 : Inport  Port=2
  T3 : Inport  Port=3
  EB3 : Inport  Port=4
  Control : Subsystem
  Memory : Memory
  TankModel : Subsystem
  LL3 : Outport
  wires:
  TankModel/1(LiquidLevel) -> Memory/1, LL3/1
  Control/2(LiquidOut) -> TankModel/2(LiquidOut)
  Memory/1 -> Control/5(LiquidLevel)
  MR3/1 -> Control/2(ManualReference)
  CT3/1 -> Control/1(ControlType)
  EB3/1 -> Control/3(EmergencyButton)
  T3/1 -> Control/4(Temperature)
  Control/1(LiquidIn) -> TankModel/1(LiquidIn)

== system c00002M_harness/M242/Tank1 ==
  CT1 : Inport
  MR1 : Inport  Port=2
  T1 : Inport  Port=3
  EB1 : Inport  Port=4
  Control : Subsystem
  Memory : Memory
  TankModel : Subsystem
  LL1 : Outport
  wires:
  TankModel/1(LiquidLevel) -> Memory/1, LL1/1
  Control/2(LiquidOut) -> TankModel/2(LiquidOut)
  Memory/1 -> Control/5(LiquidLevel)
  MR1/1 -> Control/2(ManualReference)
  CT1/1 -> Control/1(ControlType)
  EB1/1 -> Control/3(EmergencyButton)
  T1/1 -> Control/4(Temperature)
  Control/1(LiquidIn) -> TankModel/1(LiquidIn)

== system c00002M_harness/M242/Tank3 ==
  CT3 : Inport
  MR3 : Inport  Port=2
  T3 : Inport  Port=3
  EB3 : Inport  Port=4
  Control : Subsystem
  Memory : Memory
  TankModel : Subsystem
  LL3 : Outport
  wires:
  TankModel/1(LiquidLevel) -> Memory/1, LL3/1
  Control/2(LiquidOut) -> TankModel/2(LiquidOut)
  Memory/1 -> Control/5(LiquidLevel)
  MR3/1 -> Control/2(ManualReference)
  CT3/1 -> Control/1(ControlType)
  EB3/1 -> Control/3(EmergencyButton)
  T3/1 -> Control/4(Temperature)
  Control/1(LiquidIn) -> TankModel/1(LiquidIn)

== system c00002M_harness/M243/Tank1 ==
  CT1 : Inport
  MR1 : Inport  Port=2
  T1 : Inport  Port=3
  EB1 : Inport  Port=4
  Control : Subsystem
  Memory : Memory
  TankModel : Subsystem
  LL1 : Outport
  wires:
  TankModel/1(LiquidLevel) -> Memory/1, LL1/1
  Control/2(LiquidOut) -> TankModel/2(LiquidOut)
  Memory/1 -> Control/5(LiquidLevel)
  MR1/1 -> Control/2(ManualReference)
  CT1/1 -> Control/1(ControlType)
  EB1/1 -> Control/3(EmergencyButton)
  T1/1 -> Control/4(Temperature)
  Control/1(LiquidIn) -> TankModel/1(LiquidIn)

== system c00002M_harness/M243/Tank3 ==
  CT3 : Inport
  MR3 : Inport  Port=2
  T3 : Inport  Port=3
  EB3 : Inport  Port=4
  Control : Subsystem
  Memory : Memory
  TankModel : Subsystem
  LL3 : Outport
  wires:
  TankModel/1(LiquidLevel) -> Memory/1, LL3/1
  Control/2(LiquidOut) -> TankModel/2(LiquidOut)
  Memory/1 -> Control/5(LiquidLevel)
  MR3/1 -> Control/2(ManualReference)
  CT3/1 -> Control/1(ControlType)
  EB3/1 -> Control/3(EmergencyButton)
  T3/1 -> Control/4(Temperature)
  Control/1(LiquidIn) -> TankModel/1(LiquidIn)

== system c00002M_harness/M244/Tank1 ==
  CT1 : Inport
  MR1 : Inport  Port=2
  T1 : Inport  Port=3
  EB1 : Inport  Port=4
  Control : Subsystem
  Memory : Memory
  TankModel : Subsystem
  LL1 : Outport
  wires:
  TankModel/1(LiquidLevel) -> Memory/1, LL1/1
  Control/2(LiquidOut) -> TankModel/2(LiquidOut)
  Memory/1 -> Control/5(LiquidLevel)
  MR1/1 -> Control/2(ManualReference)
  CT1/1 -> Control/1(ControlType)
  EB1/1 -> Control/3(EmergencyButton)
  T1/1 -> Control/4(Temperature)
  Control/1(LiquidIn) -> TankModel/1(LiquidIn)

== system c00002M_harness/M244/Tank3 ==
  CT3 : Inport
  MR3 : Inport  Port=2
  T3 : Inport  Port=3
  EB3 : Inport  Port=4
  Control : Subsystem
  Memory : Memory
  TankModel : Subsystem
  LL3 : Outport
  wires:
  TankModel/1(LiquidLevel) -> Memory/1, LL3/1
  Control/2(LiquidOut) -> TankModel/2(LiquidOut)
  Memory/1 -> Control/5(LiquidLevel)
  MR3/1 -> Control/2(ManualReference)
  CT3/1 -> Control/1(ControlType)
  EB3/1 -> Control/3(EmergencyButton)
  T3/1 -> Control/4(Temperature)
  Control/1(LiquidIn) -> TankModel/1(LiquidIn)

== system c00002M_harness/M245/Tank1 ==
  CT1 : Inport
  MR1 : Inport  Port=2
  T1 : Inport  Port=3
  EB1 : Inport  Port=4
  Control : Subsystem
  Memory : Memory
  TankModel : Subsystem
  LL1 : Outport
  wires:
  TankModel/1(LiquidLevel) -> Memory/1, LL1/1
  Control/2(LiquidOut) -> TankModel/2(LiquidOut)
  Memory/1 -> Control/5(LiquidLevel)
  MR1/1 -> Control/2(ManualReference)
  CT1/1 -> Control/1(ControlType)
  EB1/1 -> Control/3(EmergencyButton)
  T1/1 -> Control/4(Temperature)
  Control/1(LiquidIn) -> TankModel/1(LiquidIn)

== system c00002M_harness/M245/Tank3 ==
  CT3 : Inport
  MR3 : Inport  Port=2
  T3 : Inport  Port=3
  EB3 : Inport  Port=4
  Control : Subsystem
  Memory : Memory
  TankModel : Subsystem
  LL3 : Outport
  wires:
  TankModel/1(LiquidLevel) -> Memory/1, LL3/1
  Control/2(LiquidOut) -> TankModel/2(LiquidOut)
  Memory/1 -> Control/5(LiquidLevel)
  MR3/1 -> Control/2(ManualReference)
  CT3/1 -> Control/1(ControlType)
  EB3/1 -> Control/3(EmergencyButton)
  T3/1 -> Control/4(Temperature)
  Control/1(LiquidIn) -> TankModel/1(LiquidIn)

== system c00002M_harness/M246/Tank1 ==
  CT1 : Inport
  MR1 : Inport  Port=2
  T1 : Inport  Port=3
  EB1 : Inport  Port=4
  Control : Subsystem
  Memory : Memory
  TankModel : Subsystem
  LL1 : Outport
  wires:
  TankModel/1(LiquidLevel) -> Memory/1, LL1/1
  Control/2(LiquidOut) -> TankModel/2(LiquidOut)
  Memory/1 -> Control/5(LiquidLevel)
  MR1/1 -> Control/2(ManualReference)
  CT1/1 -> Control/1(ControlType)
  EB1/1 -> Control/3(EmergencyButton)
  T1/1 -> Control/4(Temperature)
  Control/1(LiquidIn) -> TankModel/1(LiquidIn)

== system c00002M_harness/M246/Tank3 ==
  CT3 : Inport
  MR3 : Inport  Port=2
  T3 : Inport  Port=3
  EB3 : Inport  Port=4
  Control : Subsystem
  Memory : Memory
  TankModel : Subsystem
  LL3 : Outport
  wires:
  TankModel/1(LiquidLevel) -> Memory/1, LL3/1
  Control/2(LiquidOut) -> TankModel/2(LiquidOut)
  Memory/1 -> Control/5(LiquidLevel)
  MR3/1 -> Control/2(ManualReference)
  CT3/1 -> Control/1(ControlType)
  EB3/1 -> Control/3(EmergencyButton)
  T3/1 -> Control/4(Temperature)
  Control/1(LiquidIn) -> TankModel/1(LiquidIn)

== system c00002M_harness/CPSUT/Tank1/Control ==
  note: 1: Maintenance
      | 2: Reference
      | 3: Manual
  ControlType : Inport
  ManualReference : Inport  Port=2
  EmergencyButton : Inport  Port=3
  Temperature : Inport  Port=4
  LiquidLevel : Inport  Port=5
  Constant : Constant  Value=0
  Constant1 : Constant  Value=TempThreshold
  Logical Operator : Logic  Operator=OR  AllPortsSameDT=off  OutDataTypeStr=boolean
  Logical Operator1 : Logic  Operator=OR  AllPortsSameDT=off  OutDataTypeStr=boolean
  ManualControlReference : Subsystem
  Relational Operator : RelationalOperator  Operator=>  OutDataTypeStr=boolean  RndMeth=Simplest
  Switch : Switch  Criteria=u2 > Threshold
  Switch1 : Switch  Criteria=u2 > Threshold
  LiquidIn : Outport
  LiquidOut : Outport  Port=2
  wires:
  ManualReference/1 -> ManualControlReference/1(ManualReference)
  LiquidLevel/1 -> ManualControlReference/2(LiquidLevel)
  Switch/1 -> LiquidIn/1
  Switch1/1 -> LiquidOut/1
  Constant/1 -> Switch1/1, Switch/1
  EmergencyButton/1 -> Logical Operator/1, Logical Operator1/1
  Relational Operator/1 -> Logical Operator1/2, Logical Operator/2
  Logical Operator/1 -> Switch1/2
  Logical Operator1/1 -> Switch/2
  Temperature/1 -> Relational Operator/1
  Constant1/1 -> Relational Operator/2
  ManualControlReference/1(LiquidIn) -> Switch/3
  ManualControlReference/2(LiquidOut) -> Switch1/3

== system c00002M_harness/CPSUT/Tank1/TankModel ==
  LiquidIn : Inport
  LiquidOut : Inport  Port=2
  Add1 : Sum  Inputs=+-
  Constant1 : Constant  Value=0
  Constant2 : Constant  Value=0
  Constant3 : Constant
  Gain : Gain  Gain=1/R1
  Gain1 : Gain  Gain=1/A1
  Gain2 : Gain  Gain=1/R2
  Integrator : Integrator
  Saturation : Saturate  UpperLimit=hmax  LowerLimit=0
  Switch : Switch  Criteria=u2 ~= 0
  Switch1 : Switch  Criteria=u2 ~= 0
  LiquidLevel : Outport
  wires:
  Saturation/1 -> LiquidLevel/1, Gain2/1
  LiquidOut/1 -> Switch/2
  Add1/1 -> Gain1/1
  Gain2/1 -> Switch/1
  LiquidIn/1 -> Switch1/2
  Switch/1 -> Add1/2
  Switch1/1 -> Gain/1
  Constant2/1 -> Switch/3
  Constant3/1 -> Switch1/1
  Integrator/1 -> Saturation/1
  Gain1/1 -> Integrator/1
  Gain/1 -> Add1/1
  Constant1/1 -> Switch1/3

== system c00002M_harness/CPSUT/Tank3/Control ==
  note: 1: Maintenance
      | 2: Reference
      | 3: Manual
  ControlType : Inport
  ManualReference : Inport  Port=2
  EmergencyButton : Inport  Port=3
  Temperature : Inport  Port=4
  LiquidLevel : Inport  Port=5
  Constant : Constant  Value=0
  Constant1 : Constant  Value=TempThreshold
  Logical Operator : Logic  Operator=OR  AllPortsSameDT=off  OutDataTypeStr=boolean
  Logical Operator1 : Logic  Operator=OR  AllPortsSameDT=off  OutDataTypeStr=boolean
  ManualControlReference : Subsystem
  Relational Operator : RelationalOperator  Operator=>  OutDataTypeStr=boolean  RndMeth=Simplest
  Switch : Switch  Criteria=u2 > Threshold
  Switch1 : Switch  Criteria=u2 > Threshold
  LiquidIn : Outport
  LiquidOut : Outport  Port=2
  wires:
  ManualReference/1 -> ManualControlReference/1(ManualReference)
  LiquidLevel/1 -> ManualControlReference/2(LiquidLevel)
  Switch/1 -> LiquidIn/1
  Switch1/1 -> LiquidOut/1
  Constant/1 -> Switch1/1, Switch/1
  EmergencyButton/1 -> Logical Operator/1, Logical Operator1/1
  Relational Operator/1 -> Logical Operator1/2, Logical Operator/2
  Logical Operator/1 -> Switch1/2
  Logical Operator1/1 -> Switch/2
  Temperature/1 -> Relational Operator/1
  Constant1/1 -> Relational Operator/2
  ManualControlReference/1(LiquidIn) -> Switch/3
  ManualControlReference/2(LiquidOut) -> Switch1/3

== system c00002M_harness/CPSUT/Tank3/TankModel ==
  LiquidIn : Inport
  LiquidOut : Inport  Port=2
  Add1 : Sum  Inputs=+-
  Constant1 : Constant  Value=0
  Constant2 : Constant  Value=0
  Constant3 : Constant
  Gain : Gain  Gain=1/R1
  Gain1 : Gain  Gain=1/A1
  Gain2 : Gain  Gain=1/R2
  Integrator : Integrator
  Saturation : Saturate  UpperLimit=hmax  LowerLimit=0
  Switch : Switch  Criteria=u2 ~= 0
  Switch1 : Switch  Criteria=u2 ~= 0
  LiquidLevel : Outport
  wires:
  Saturation/1 -> LiquidLevel/1, Gain2/1
  LiquidOut/1 -> Switch/2
  Add1/1 -> Gain1/1
  Gain2/1 -> Switch/1
  LiquidIn/1 -> Switch1/2
  Switch/1 -> Add1/2
  Switch1/1 -> Gain/1
  Constant2/1 -> Switch/3
  Constant3/1 -> Switch1/1
  Integrator/1 -> Saturation/1
  Gain1/1 -> Integrator/1
  Gain/1 -> Add1/1
  Constant1/1 -> Switch1/3
